simulink model "part1"  (R2018a)
settings: Solver=VariableStepAuto  StartTime=0.0  StopTime=1.0  RelTol=1e-3
libraries: truetime x4
settings Model: Creator=Ismael  LastModifiedBy=Ismael

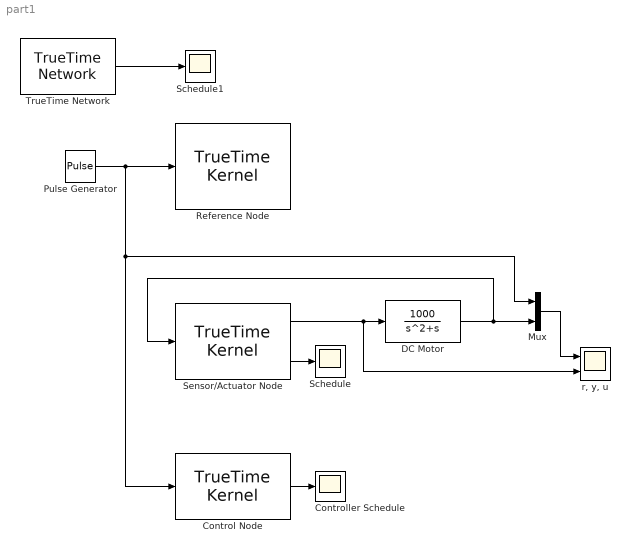
== system part1 ==
  "Control Node " : truetime/TrueTime Kernel  sfun=control_init  args=0  ninputsoutputs=[1 0]  ntriggers=0  trigtype=rising  nwnodenbr=3  clockoffsetdrift=[0 0]  schedoutput=on  battery=off  poweroutput=off  label=1: 3
  Controller Schedule : Scope
  DC Motor : TransferFcn  Numerator=[1000]  Denominator=[1 1 0]
  Mux : Mux  Inputs=2
  "Pulse Generator " : DiscretePulseGenerator  PulseType=Time based  Amplitude=2  Period=1  PulseWidth=50  PhaseDelay=0.1
  "Reference Node " : truetime/TrueTime Kernel  sfun=reference_init  args=0  ninputsoutputs=[1 0]  ntriggers=0  trigtype=rising  nwnodenbr=1  clockoffsetdrift=[0 0]  schedoutput=off  battery=off  poweroutput=off  label=1: 1
  Schedule : Scope
  Schedule1 : Scope
  "Sensor/Actuator Node " : truetime/TrueTime Kernel  sfun=sens_act_init  args=0  ninputsoutputs=[1 1]  ntriggers=0  trigtype=falling  nwnodenbr=2  clockoffsetdrift=[0 0]  schedoutput=on  battery=off  poweroutput=off  label=1: 2
  TrueTime Network : truetime/TrueTime Network  nwtype=CSMA/AMP (CAN)  nwnbr=1  nnodes=3  rate=80000  minsize=40  lossprob=0  seed=0  bandwidths=[0.5 0.5]  slotsize=512  schedule=[1 1 2]  memsize=80000  buftype=Common buffer  overflow=Retransmit  dynSchedule=0  miniSlotSize=0  NIT=0  QSortMode=FIFO  sync=0  irtSchedule=0  nrtLength=0  nodeGraph=0  scheduleoutput=on
  "r, y, u " : Scope  NumInputPorts=2
  wires:
  "Sensor/Actuator Node "/1 -> "r, y, u "/2, DC Motor/1
  "Sensor/Actuator Node "/2 -> Schedule/1
  DC Motor/1 -> "Sensor/Actuator Node "/1, Mux/2
  Mux/1 -> "r, y, u "/1
  "Control Node "/1 -> Controller Schedule/1
  TrueTime Network/1 -> Schedule1/1
  "Pulse Generator "/1 -> "Control Node "/1, Mux/1, "Reference Node "/1
